simulink model "simplified_generator"  (R2022a)
settings: Solver=VariableStepAuto  StartTime=0.0  StopTime=10.0  RelTol=1e-3
values from neighbouring files (symbols this model uses):
  B_eq = param{6}    [measurement_2states.m]    (also in measurement_2states_3mes.m; measurement_3measure.m)
undefined symbols (not defined in the file or in its folder): Gc, generator, I_eq, rotor, simulation
libraries: simulink x1
settings Model: Creator=Niccolò  LastModifiedBy=Niccolò

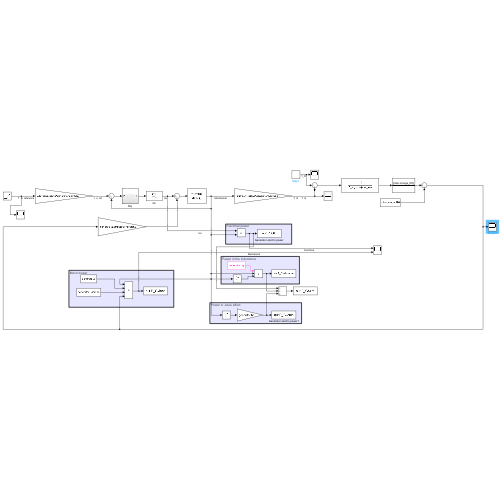
[thumbnail: Simulink's stored preview of the top-level diagram]
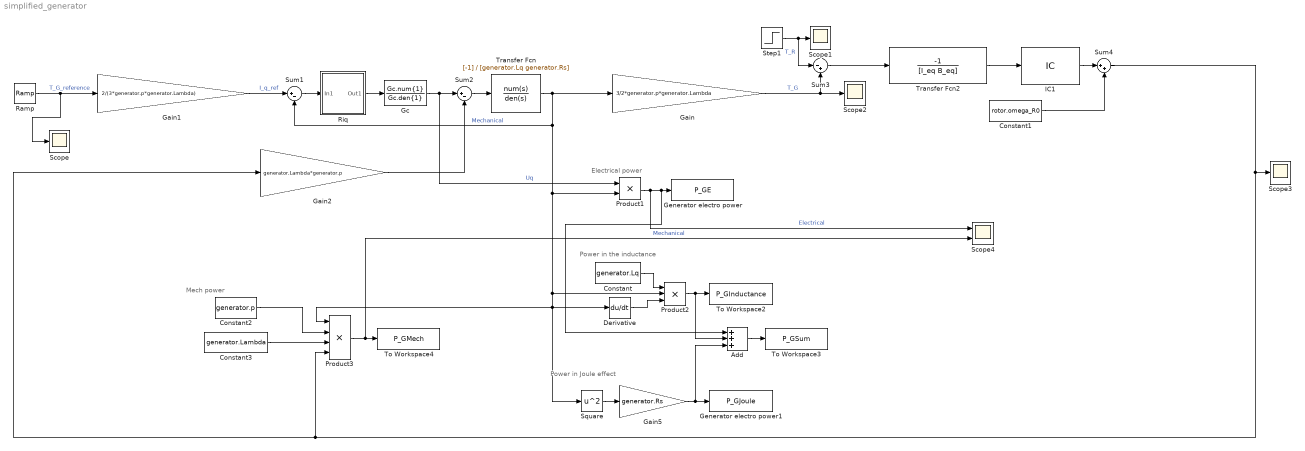
== system simplified_generator ==
  note: Mech power
  note: Power in Joule effect
  note: Power in the inductance
  note: Electrical power
  Add : Sum  Inputs=3
  Constant : Constant  Value=generator.Lq
  Constant1 : Constant  Value=rotor.omega_R0
  Constant2 : Constant  Value=generator.p
  Constant3 : Constant  Value=generator.Lambda
  Derivative : Derivative
  Gain : Gain  Gain=3/2*generator.p*generator.Lambda  SampleTime=simulation.time_step_L
  Gain1 : Gain  Gain=2/(3*generator.p*generator.Lambda)  SampleTime=simulation.time_step_L
  Gain2 : Gain  Gain=generator.Lambda*generator.p
  Gain5 : Gain  Gain=generator.Rs
  Gc : TransferFcn  Numerator=Gc.num{1}  Denominator=Gc.den{1}
  Generator electro power : ToWorkspace  VariableName=P_GE  SaveFormat=Timeseries  SampleTime=-1
  Generator electro power1 : ToWorkspace  VariableName=P_GJoule  SaveFormat=Timeseries  SampleTime=-1
  IC1 : InitialCondition  Value=rotor.omega_R0
  Product1 : Product
  Product2 : Product  Inputs=3
  Product3 : Product  Inputs=4
  Ramp : simulink/Sources/Ramp  slope=1e5  start=0  InitialOutput=0
  Riq : Subsystem
  Scope{,1..3} (4 alike) : Scope
  Scope4 : Scope  NumInputPorts=2
  Square : Math  Operator=square
  Step1 : Step  Time=0  After=0  SampleTime=0
  Sum1 : Sum  Inputs=|+-  SampleTime=simulation.time_step_L
  Sum2 : Sum  Inputs=|+-
  Sum3 : Sum  Inputs=|-+
  Sum4 : Sum  Inputs=|++
  To Workspace2 : ToWorkspace  VariableName=P_GInductance  SaveFormat=Timeseries  SampleTime=-1
  To Workspace3 : ToWorkspace  VariableName=P_GSum  SaveFormat=Timeseries  SampleTime=-1
  To Workspace4 : ToWorkspace  VariableName=P_GMech  SaveFormat=Timeseries  SampleTime=-1
  Transfer Fcn : TransferFcn  Numerator=[-1]  Denominator=[generator.Lq generator.Rs]
  Transfer Fcn2 : TransferFcn  Numerator=[-1]  Denominator=[I_eq B_eq]
  wires:
  Sum4/1 -> Gain2/1, Product3/4, Scope3/1
  Product2/1 -> To Workspace2/1, Add/2
  Derivative/1 -> Product2/3
  Constant3/1 -> Product3/3
  Sum2/1 -> Transfer Fcn/1
  Product1/1 -> Scope4/1, Add/1, Generator electro power/1  "Electrical"
  Gain5/1 -> Add/3, Generator electro power1/1
  Constant2/1 -> Product3/2
  Constant/1 -> Product2/1
  Gain2/1 -> Sum2/2
  Square/1 -> Gain5/1
  Ramp/1 -> Gain1/1, Scope/1  "T_G_reference"
  Product3/1 -> Scope4/2, To Workspace4/1  "Mechanical"
  Riq/1(Out1) -> Gc/1
  Gc/1 -> Product1/1, Sum2/1  "Uq"
  Gain/1 -> Scope2/1, Sum3/2  "T_G"
  Transfer Fcn/1 -> Gain/1, Sum1/2, Product1/2, Product3/1, Square/1, Derivative/1, Product2/2  "Mechanical"
  Sum1/1 -> Riq/1(In1)
  Add/1 -> To Workspace3/1
  Gain1/1 -> Sum1/1  "I_q_ref"
  Constant1/1 -> Sum4/2
  Sum3/1 -> Transfer Fcn2/1
  Transfer Fcn2/1 -> IC1/1
  Step1/1 -> Sum3/1, Scope1/1  "T_R"
  IC1/1 -> Sum4/1

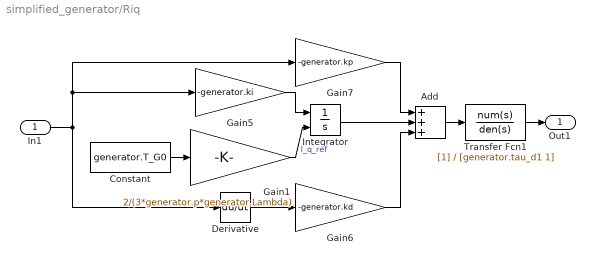
== system simplified_generator/Riq ==
  In1 : Inport
  Add : Sum  Inputs=+++
  Constant : Constant  Value=generator.T_G0
  Derivative : Derivative
  Gain1 : Gain  Gain=2/(3*generator.p*generator.Lambda)  SampleTime=simulation.time_step_L
  Gain5 : Gain  Gain=-generator.ki
  Gain6 : Gain  Gain=-generator.kd
  Gain7 : Gain  Gain=-generator.kp
  Integrator : Integrator  InitialConditionSource=external
  Transfer Fcn1 : TransferFcn  Denominator=[generator.tau_d1 1]
  Out1 : Outport
  wires:
  Integrator/1 -> Add/2
  Add/1 -> Transfer Fcn1/1
  Constant/1 -> Gain1/1
  Gain7/1 -> Add/1
  Gain6/1 -> Add/3
  Derivative/1 -> Gain6/1
  In1/1 -> Gain5/1, Gain7/1, Derivative/1
  Transfer Fcn1/1 -> Out1/1
  Gain5/1 -> Integrator/1
  Gain1/1 -> Integrator/2  "I_q_ref"
